simulink model "power_PVarray_grid_det"  (R2016a)
settings: Solver=FixedStepDiscrete  SolverMode=SingleTasking  StartTime=0.0  StopTime=2.5  RelTol=1e-3
PreLoadFcn:
  | Ts_Power=1e-6;
  | Ts_Control=100e-6;
undefined symbols (not defined in the file): D1, Delta, DiscIntNeverNeededParam, sigbuilder_block
libraries: powerlib x23, powerlib_meascontrol x11, simulink x2, re_lib x1
(part 1 of 2)
Description:
  | Copyright 2008-2016 The MathWorks, Inc.
settings Model: SimulationMode=accelerator  Creator=MathWorks  LastModifiedBy=mesutto
settings DataIOCC: LimitDataPoints=on  SaveFormat=Array  SignalLoggingSaveFormat=ModelDataLogs  SignalLogging=off  DSMLogging=off
settings OptimizationCC: ExpressionDepthLimit=2147483647
settings DebuggingCC: UnderspecifiedInitializationDetection=Classic  MergeDetectMultiDrivingBlocksExec=none  SolverPrmCheckMsg=warning  FcnCallInpInsideContextMsg=UseLocalSettings  StateNameClashWarn=warning
settings HardwareCC: ProdBitPerPointer=32  ProdLargestAtomicFloat=None  ProdIntDivRoundTo=Undefined  ProdEndianess=Unspecified  ProdWordSize=32  ProdHWDeviceType=32-bit Generic
settings ModelReferenceCC: PropagateSignalLabelsOutOfModel=off
settings GRTTargetCC: CombineOutputUpdateFcns=off  GRTInterface=on
settings ConfigComp: CovModelRefEnable=Off  CovSFcnEnable=off

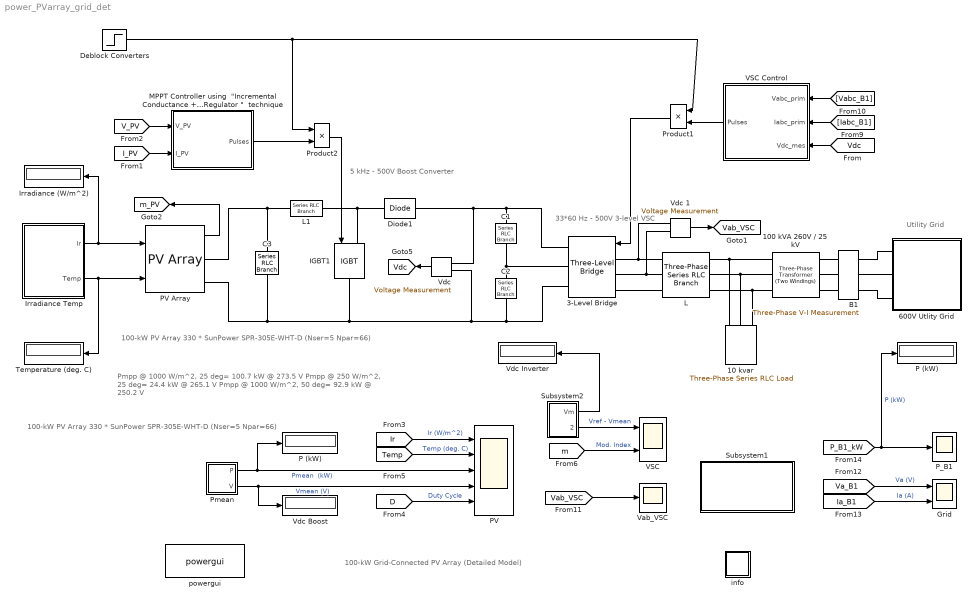
== system power_PVarray_grid_det ==
  note: 5 kHz - 500V
      | Boost Converter
  note: 33*60 Hz - 500V
      | 3-level VSC
  note: 100-kW Grid-Connected PV Array (Detailed Model)
  note: Utility Grid
  note: Pmpp @ 1000 W/m^2, 25 deg= 100.7 kW @ 273.5 V
      | Pmpp @  250 W/m^2, 25 deg= 24.4  kW @ 265.1 V
      | Pmpp @ 1000 W/m^2, 50 deg= 92.9  kW @ 250.2 V
  note: 100-kW  PV Array
      | 330 * SunPower SPR-305E-WHT-D  (Nser=5 Npar=66)
  note: 100-kW  PV Array
      | 330 * SunPower SPR-305E-WHT-D  (Nser=5 Npar=66)
  10 kvar : powerlib/Elements/Three-Phase Series RLC Load  LConnTagsString=A|B|C  Configuration=Y (grounded)  NominalVoltage=240  Vabc=[1e3 1e3 1e3]  Vabcp=[1e3 1e3 1e3]  NominalFrequency=60  UnbalancedPower=off  ActivePower=10e3/100  InductivePower=0  CapacitivePower=10e3  Pabc=[10e3 9e3 11e3]  QLabc=[100 90 110]  QCabc=[100 90 110]  Pabcp=[10e3 9e3 11e3]  QLabcp=[100 90 110]  QCabcp=[100 90 110]  Measurements=None  LoadType=constant Z
  100 kVA 260V / 25 kV : powerlib/Elements/Three-Phase Transformer (Two Windings)  Winding1Connection=Yg  Winding2Connection=Delta (D1)  CoreType=Three single-phase transformers  SetSaturation=off  Hysteresis=off  DataFile='hysteresis'  SetInitialFlux=off  Measurements=None  UNITS=pu  NominalPower=[100e3 , 60 ]  Winding1=[ 25e3 , 0.001 , 0.03 ]  Winding2=[ 260 , 0.001 , 0.03 ]  Rm=500  Lm=500  L0=0.5  Saturation=[ 0,0 ; 0.0024,1.2 ; 1.0,1.52 ]  InitialFluxes=[ 0.8 , -0.8 , 0.7 ]  MoreParameters=off  BreakLoop=off  DataType=off  TransfoNumber=0
  3-Level Bridge : powerlib/Power Electronics/Three-Level Bridge  Arms=3  SnubberResistance=1e6  SbubberCapacitance=inf  Device=IGBT / Diodes  Ron=0.2e-3  ForwardVoltages="[  0  0 ]"  Measurements=None
  600V Utlity Grid : Subsystem
      mask Display: image(imread('grid.jpg'))
  B1 : powerlib/Measurements/Three-Phase V-I Measurement  VoltageMeasurement=phase-to-ground  SetLabelV=on  LabelV=Vabc_B1  Vpu=off  VpuLL=off  CurrentMeasurement=yes  SetLabelI=on  LabelI=Iabc_B1  Ipu=off  Pbase=100e6  Vbase=500e3  OutputType=Magnitude  PhasorSimulation=off  PSBequivalent=0
  C1 : powerlib/Elements/Series RLC Branch  LConnTagsString=__new0  RConnTagsString=__new0  BranchType=C  Resistance=1.0  Inductance=1.0  SetiL0=off  InitialCurrent=0  Capacitance=12000e-06  Setx0=off  InitialVoltage=0  Measurements=None
  C2 : powerlib/Elements/Series RLC Branch  LConnTagsString=__new0  RConnTagsString=__new0  BranchType=C  Resistance=1.0  Inductance=1.0  SetiL0=off  InitialCurrent=0  Capacitance=12000e-06  Setx0=off  InitialVoltage=0  Measurements=None
  C3 : powerlib/Elements/Series RLC Branch  LConnTagsString=__new0  RConnTagsString=__new0  BranchType=C  Resistance=1.0  Inductance=1.0  SetiL0=off  InitialCurrent=0  Capacitance=100e-6  Setx0=off  InitialVoltage=0  Measurements=Branch voltage
  Deblock Converters : Step  Time=0.05  SampleTime=0
  Diode1 : powerlib/Power Electronics/Diode  Ron=1e-4  Lon=0  Vf=0  IC=0  UseSnubber=off  Rs=inf  Cs=inf  Measurements=off
  Grid : Scope  NumInputPorts=2
  IGBT1 : powerlib/Power Electronics/IGBT  Ron=0.001  Lon=0  Vf=0  Tf=0  Tt=0  IC=0  Rs=1e5  Cs=inf  Measurements=off
  Irradiance (W/m^2) : Display
      settings: Format=bank  Decimation=1000
  Irradiance Temp : Subsystem  Tag=STV Subsys  LoadFcn=sigbuilder_block('load');  StartFcn=sigbuilder_block('start');  StopFcn=sigbuilder_block('stop');  ClipboardFcn=sigbuilder_block('clipboard');  mask(Sigbuilder block){}
      mask help: Sigbuilder GUI
      mask init:
      | if ~strcmp(get_param(bdroot(gcbh),'SimulationStatus'),'stopped') tuvar = sigbuilder_block('maskInit'); end
      settings: CopyFcn=sigbuilder_block('copy');  DeleteFcn=sigbuilder_block('delete');  ModelCloseFcn=sigbuilder_block('modelClose');  PreSaveFcn=sigbuilder_block('preSave');  PauseFcn=sigbuilder_block('pause')  ContinueFcn=sigbuilder_block('continue')  NameChangeFcn=sigbuilder_block('namechange');  OpenFcn=sigbuilder_block('open',[216.75 153.75 550.5 395.25 ]);  CloseFcn=sigbuilder_block('close');
      mask Display: plot(0,0,100,100,[10,10,40,40,10],[80,20,20,80,80],[40,10],[50,50], [40,27,10],[65,72,56],[40,25,25,10],[28,28,43,43]);
  L : powerlib/Elements/Three-Phase Series RLC Branch  LConnTagsString=A|B|C  RConnTagsString=A|B|C  BranchType=RL  Resistance=500e-6*377/50/2  Inductance=500e-6/2  Capacitance=inf  Measurements=None
  L1 : powerlib/Elements/Series RLC Branch  LConnTagsString=__new0  RConnTagsString=__new0  BranchType=RL  Resistance=0.005  Inductance=5e-3  SetiL0=off  InitialCurrent=0  Capacitance=1e-6  Setx0=off  InitialVoltage=0  Measurements=None
  "MPPT Controller using  \"Incremental Conductance + Integral Regulator \"  technique " : Subsystem  mask(Boost Control - MPPT){fc=5000, T_MPPT=200e-6, Dinit=0.5}
      mask prompts: fc "PWM switching frequency (Hz)"; T_MPPT "Time window used by MPPT control (s)"; Dinit "Initial value of duty cycle"
  P (kW) : Display
      settings: Format=bank  Decimation=2000
  "P (kW) " : Display
      settings: Format=bank  Decimation=2000
  PV : Scope  NumInputPorts=5
  PV Array : re_lib/Solar/PV Array  Npar=66  Nser=5  PlotType=array @ 1000 W/m2 & specified temperatures  S_vec="[ 1000  250 ]"  Temp_C_vec="[0 25 50  ]"  ModuleName=SunPower SPR-305E-WHT-D  PlotWhenSelected=off  Pm=305.226  Ncell=96  Voc=64.2  Isc=5.96  Vm=54.7  Im=5.58  beta_Voc_pc=-0.27269  alpha_Isc_pc=0.061745  beta_Voc=-0.17507  alpha_Isc=0.00368  IL=6.0092  I0=6.3014e-12  nI=0.94504  Rsh=269.5934  Rs=0.37152  BAL=on  Tc=Tc  Tfilter=5e-5
  P_B1 : Scope
  Pmean : Subsystem
  Product1 : Product  RndMeth=Zero
  Product2 : Product  RndMeth=Zero
  Subsystem1 : Subsystem
      mask Display: disp('Open this block\nto display additional \nscopes & measurements')
  Subsystem2 : Subsystem
  Temperature (deg. C) : Display
      settings: Format=bank  Decimation=1000
  VSC : Scope  NumInputPorts=2
  VSC Control : Subsystem  mask(VSC Main Controller){nom=[ 100e3  60 ], Vnom=[ 25e3 260 ], Vnom_dc=500, RLxfo=[0.002  0.06 ], RLchoke=[2e-3  250e-6  ], K_VDCreg=[7  800], K_Ireg=[0.3 20], Ts=Ts_Control}
      mask prompts: nom "Nominal power and frequency [ Pnom(VA)  Fnom(Hz) ]:"; Vnom "Nominal primary and secondary voltages (Vrms LL) [ Vnom_prim   Vnom_sec ]:"; Vnom_dc "Nominal DC bus voltage (V):"; RLxfo "Total transformer leakage impedance (pu/Pnom) [ Rxfo  Lxf ]"; RLchoke "Choke impedance [ R(ohm) L(H) ]"; K_VDCreg "VDC regultator gains [ Kp  Ki ]:"; K_Ireg "Current regulator gains [ Kp  Ki ]:"; Ts "Sample time"
      mask init:
      | Pnom=nom(1);
      | Fnom=nom(2);
      | Vnom_prim=Vnom(1);
      | Vnom_sec=Vnom(2);
      | Zbase=Vnom_sec^2/Pnom;
      | Rtot_pu=RLxfo(1) + RLchoke(1)/Zbase;
      | Ltot_pu=RLxfo(2) + RLchoke(2)/(Zbase/(2*pi*Fnom));
      | Kp_VDCreg=K_VDCreg(1);
      | Ki_VDCreg=K_VDCreg(2);
      | Kp_Ireg=K_Ireg(1);
      | Ki_Ireg=K_Ireg(2);
      | Vdc_ref=Vnom_dc;
      | % Used to determine initial value of Boost Control (MPPT)
      | assignin('base','Vdc_ref_Inv',Vdc_ref);
  Vab_VSC : Scope
  "Vdc " : powerlib/Measurements/Voltage Measurement  Tag=PoWeRsYsTeMmEaSuReMeNt  PhasorSimulation=off  OutputType=Magnitude  PSBequivalent=0
  Vdc 1 : powerlib/Measurements/Voltage Measurement  Tag=PoWeRsYsTeMmEaSuReMeNt  PhasorSimulation=off  OutputType=Magnitude  PSBequivalent=0
  Vdc Boost : Display
      settings: Format=bank  Decimation=2000
  Vdc Inverter : Display
      settings: Format=bank  Decimation=2000
  info : Subsystem
      settings: OpenFcn=showdemo(bdroot(gcb))
      mask Display: disp('?')
  powergui : powerlib/powergui  Priority=1  SimulationMode=Discrete  SolverType=Tustin/Backward Euler (TBE)  SampleTime=Ts_Power  frequency=60  SPID=off  DisableSnubberDevices=off  DisableRonSwitches=off  DisableVfSwitches=off  SwTol=0  DisplayEquations=off  Interpol=off  ExternalGateDelay=off  methode=off  Ts=0  FunctionMessages=off  echomessages=off  HookPort=off  EnableUseOfTLC=off  x0status=blocks  frequencyindice=0  Pbase=100e6  ErrMax=1e-4  Iterations=50  UnitsV=kV  UnitsW=MW  buscounter=0  RestoreLinks=warning  ResistiveCurrentMeasurement=off  Frange=[0:2:500]  Ylog=off  Xlog=on  ShowGrid=off  save=off  variable=ZData  structure=0  ZoomFFT=on  StartTime=0.0  cycles=1  DisplayStyle=1  fundamental=60  FreqAxis=off  MaxFrequency=1000  frequencyindicesteady=1  RmsSteady=1  display=off
  tag scope: Vab_VSC=global, Vdc=global, m_PV=global
  wires:
  "Vdc "/1 -> [Vdc]
  Product2/1 -> IGBT1/1
  "MPPT Controller using  \"Incremental Conductance + Integral Regulator \"  technique "/1(Pulses) -> Product2/2
  Deblock Converters/1 -> Product2/1, Product1/1
  [Vabc_B1] -> VSC Control/1(Vabc_prim)
  [Iabc_B1] -> VSC Control/2(Iabc_prim)
  [Vdc] -> VSC Control/3(Vdc_mes)
  VSC Control/1(Pulses) -> Product1/2
  Product1/1 -> 3-Level Bridge/1
  [I_PV] -> "MPPT Controller using  \"Incremental Conductance + Integral Regulator \"  technique "/2(I_PV)
  [V_PV] -> "MPPT Controller using  \"Incremental Conductance + Integral Regulator \"  technique "/1(V_PV)
  Pmean/1(P) -> "P (kW) "/1, PV/3  "Pmean  (kW)"
  [m] -> VSC/2  "Mod. Index"
  Vdc 1/1 -> [Vab_VSC]
  [Vab_VSC] -> Vab_VSC/1
  [Ia_B1] -> Grid/2  "Ia (A)"
  [Va_B1] -> Grid/1  "Va (V)"
  [P_B1_kW] -> P_B1/1, P (kW)/1  "P (kW)"
  Pmean/2(V) -> Vdc Boost/1, PV/4  "Vmean (V)"
  Subsystem2/2(VrVm) -> VSC/1  "Vref - Vmean"
  Subsystem2/1(Vm) -> Vdc Inverter/1
  PV Array/1 -> [m_PV]
  Irradiance Temp/1(Ir) -> PV Array/1, Irradiance (W/m^2)/1
  Irradiance Temp/2(Temp) -> PV Array/2, Temperature (deg. C)/1
  [D] -> PV/5  "Duty Cycle"
  [Temp] -> PV/2  "Temp (deg. C)"
  [Ir] -> PV/1  "Ir (W/m^2)"
  connections:
  3-Level Bridge/RConn1 -- Diode1/RConn1 -- "Vdc "/LConn1 -- C1/LConn1
  L1/RConn1 -- Diode1/LConn1 -- IGBT1/LConn1
  3-Level Bridge/RConn3 -- C2/RConn1 -- "Vdc "/LConn2 -- IGBT1/RConn1 -- PV Array/RConn2 -- C3/RConn1
  3-Level Bridge/LConn1 -- L/LConn1 -- Vdc 1/LConn1
  3-Level Bridge/LConn2 -- L/LConn2 -- Vdc 1/LConn2
  3-Level Bridge/LConn3 -- L/LConn3
  L/RConn1 -- 100 kVA 260V / 25 kV/RConn1 -- 10 kvar/LConn1
  L/RConn2 -- 100 kVA 260V / 25 kV/RConn2 -- 10 kvar/LConn2
  L/RConn3 -- 100 kVA 260V / 25 kV/RConn3 -- 10 kvar/LConn3
  B1/LConn1 -- 100 kVA 260V / 25 kV/LConn1
  B1/LConn2 -- 100 kVA 260V / 25 kV/LConn2
  B1/LConn3 -- 100 kVA 260V / 25 kV/LConn3
  C2/LConn1 -- C1/RConn1 -- 3-Level Bridge/RConn2
  C3/LConn1 -- PV Array/RConn1 -- L1/LConn1
  B1/RConn2 -- 600V Utlity Grid/LConn2
  B1/RConn1 -- 600V Utlity Grid/LConn1
  B1/RConn3 -- 600V Utlity Grid/LConn3

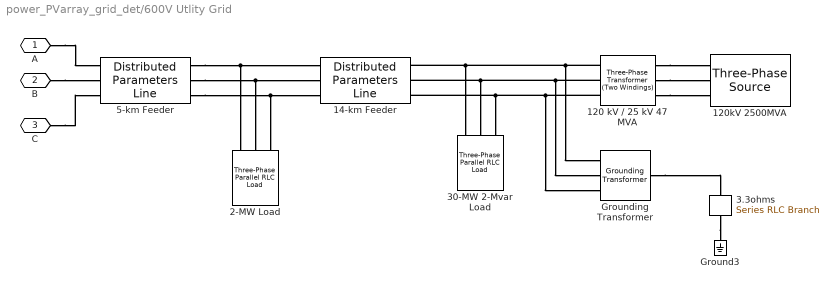
== system power_PVarray_grid_det/600V Utlity Grid ==
  120 kV / 25 kV 47 MVA : powerlib/Elements/Three-Phase Transformer (Two Windings)  Winding1Connection=Yg  Winding2Connection=Delta (D1)  CoreType=Three single-phase transformers  SetSaturation=off  Hysteresis=off  DataFile='basic_model'  SetInitialFlux=off  Measurements=None  UNITS=pu  NominalPower=[47e6 60 ]  Winding1="[ 120e3  0.08/30   0.08 ]"  Winding2="[ 25e3  0.08/30  0.08]"  Rm=500  Lm=500  L0=0.5  Saturation="[ 0,0  ;  0.005,1.2  ;  1.0,1.4 ]"  InitialFluxes=[ 0.8 , -0.8 , 0.7 ]  MoreParameters=off  BreakLoop=off  DataType=off  TransfoNumber=0
  120kV 2500MVA : powerlib/Electrical Sources/Three-Phase Source  InternalConnection=Yg  VoltagePhases=off  Voltage=120e3  PhaseAngle=0  Voltage_phases=[25e3 25e3 25e3]/sqrt(3)  PhaseAngles_phases=[0 -120 +120]  Frequency=60  NonIdealSource=on  SpecifyImpedance=on  Resistance=0.8929  Inductance=16.58e-3  ShortCircuitLevel=2500e6  BaseVoltage=120e3  XRratio=7  BusType=swing  Pref=0  Qref=0  Prefabc=[10e3, 10e3, 10e3]  Qrefabc=[0, 0, 0]  Qmin=-inf  Qmax=inf
  14-km Feeder : powerlib/Elements/Distributed Parameters Line  Phases=3  Frequency=60  Resistance=[0.1153 0.413]  Inductance=[1.05e-3 3.32e-3]  Capacitance=[11.33e-009 5.01e-009]  Length=14  x1=[-5.8e-05 -3.03124509742695e-09 0 0;-5.7e-05 -3.03083569384269e-09 0 0;-5.6e-05 -3.03042585950908e-09 0 0;-5.5e-05 -3.03001559448437e-09 0 0;-5.4e-05 -3.02960489882688e-09 0 0;-5.3e-05 -3.02919377259496e-09 0 0;-5.2e-05 -3.02878221584705e-09 0 0;-5.1e-05 -3.02837022864164e-09 0 0;-5e-05 -3.02795781103729e-09 0 0;-4.9e-05 -3.0275449630926e-09 -3790.73535189758 -24061.413420025;-4.8e-05 -3.02713168486625e-09 -3781.66414358219 -24062.8407837194;-4.7e-05 -3.02671797641698e-09 -3772.59239780798 -24064.2647275475;-4.6e-05 -3.02630383780358e-09 -3763.52011586426 -24065.6852513069;-4.5e-05 -3.02588926908492e-09 -3754.4472990404 -24067.1023547957;-4.4e-05 -3.02547427031991e-09 -3745.37394862584 -24068.5160378125;-4.3e-05 -3.02505884156753e-09 -3736.30006591012 -24069.9263001565;-4.2e-05 -3.02464298288683e-09 -3727.22565218283 -24071.3331416271;-4.1e-05 -3.0242266943369e-09 -3718.15070873366 -24072.7365620244;-4e-05 -3.02380997597692e-09 -3709.07523685235 -24074.136561149;-3.9e-05 -3.0233928278661e-09 -3699.99923782873 -24075.5331388019;-3.8e-05 -3.02297525006373e-09 -3690.9227129527 -24076.9262947847;-3.7e-05 -3.02255724262917e-09 -3681.84566351424 -24078.3160288992;-3.6e-05 -3.02213880562181e-09 -3672.7680908034 -24079.7023409481;-3.5e-05 -3.02171993910113e-09 -3663.6899961103 -24081.0852307342;-3.4e-05 -3.02130064312665e-09 -3654.61138072515 -24082.4646980611;-3.3e-05 -3.02088091775798e-09 -3645.53224593822 -24083.8407427326;-3.2e-05 -3.02046076305475e-09 -3636.45259303985 -24085.2133645533;-3.1e-05 -3.02004017907669e-09 -3627.37242332048 -24086.582563328;-3e-05 -3.01961916588357e-09 -3618.29173807058 -24087.9483388622;-2.9e-05 -3.01919772353522e-09 -3609.21053858074 -24089.3106909617;-2.8e-05 -3.01877585209154e-09 -3600.12882614158 -24090.6696194329;-2.7e-05 -3.01835355161249e-09 -3591.04660204383 -24092.0251240827;-2.6e-05 -3.01793082215809e-09 -3581.96386757827 -24093.3772047185;-2.5e-05 -3.01750766378841e-09 -3572.88062403577 -24094.725861148;-2.4e-05 -3.0170840765636e-09 -3563.79687270724 -24096.0710931796;-2.3e-05 -3.01666006054385e-09 -3554.7126148837 -24097.4129006222;-2.2e-05 -3.01623561578943e-09 -3545.62785185622 -24098.7512832849;-2.1e-05 -3.01581074236066e-09 -3536.54258491595 -24100.0862409777;-2e-05 -3.01538544031793e-09 -3527.45681535411 -24101.4177735107;-1.9e-05 -3.01495970972168e-09 -3518.37054446199 -24102.7458806947;-1.8e-05 -3.01453355063242e-09 -3509.28377353094 -24104.0705623411;-1.7e-05 -3.01410696311071e-09 -3500.19650385241 -24105.3918182614;-1.6e-05 -3.01367994721718e-09 -3491.1087367179 -24106.709648268;-1.5e-05 -3.01325250301252e-09 -3482.02047341897 -24108.0240521735;-1.4e-05 -3.01282463055748e-09 -3472.93171524728 -24109.3350297911;-1.3e-05 -3.01239632991286e-09 -3463.84246349455 -24110.6425809346;-1.2e-05 -3.01196760113955e-09 -3454.75271945255 -24111.9467054181;-1.1e-05 -3.01153844429847e-09 -3445.66248441314 -24113.2474030561;-1e-05 -3.01110885945062e-09 -3436.57175966825 -24114.544673664;-9e-06 -3.01067884665704e-09 -3427.48054650987 -24115.8385170572;-8e-06 -3.01024840597885e-09 -3418.38884623006 -24117.128933052;-7e-06 -3.00981753747724e-09 -3409.29666012097 -24118.4159214649;-6e-06 -3.00938624121342e-09 -3400.20398947478 -24119.6994821131;-5e-06 -3.00895451724871e-09 -3391.11083558378 -24120.979614814;-4e-06 -3.00852236564446e-09 -3382.0171997403 -24122.2563193858;-3e-06 -3.00808978646208e-09 -3372.92308323675 -24123.5295956469;-2e-06 -3.00765677976306e-09 -3363.82848736562 -24124.7994434166;-1e-06 -3.00722334560893e-09 -3354.73341341943 -24126.0658625142]  x2=[-5.8e-05 -3.18873630316946e-09 0 0;-5.7e-05 -3.18824656390701e-09 0 0;-5.6e-05 -3.18775637152362e-09 0 0;-5.5e-05 -3.18726572608896e-09 0 0;-5.4e-05 -3.18677462767275e-09 0 0;-5.3e-05 -3.1862830763448e-09 0 0;-5.2e-05 -3.18579107217497e-09 0 0;-5.1e-05 -3.18529861523317e-09 0 0;-5e-05 -3.18480570558941e-09 0 0;-4.9e-05 -3.18431234331373e-09 -3379.39242591108 -24244.0512732151;-4.8e-05 -3.18381852847625e-09 -3370.25239397928 -24245.323551305;-4.7e-05 -3.18332426114715e-09 -3361.11188305945 -24246.5923835937;-4.6e-05 -3.18282954139668e-09 -3351.97089445066 -24247.8577699009;-4.5e-05 -3.18233436929515e-09 -3342.82942945205 -24249.1197100467;-4.4e-05 -3.18183874491293e-09 -3333.68748936283 -24250.3782038519;-4.3e-05 -3.18134266832047e-09 -3324.54507548227 -24251.6332511374;-4.2e-05 -3.18084613958826e-09 -3315.40218910972 -24252.884851725;-4.1e-05 -3.18034915878689e-09 -3306.25883154457 -24254.1330054368;-4e-05 -3.17985172598696e-09 -3297.11500408631 -24255.3777120954;-3.9e-05 -3.1793538412592e-09 -3287.97070803447 -24256.6189715239;-3.8e-05 -3.17885550467434e-09 -3278.82594468867 -24257.8567835459;-3.7e-05 -3.17835671630323e-09 -3269.68071534858 -24259.0911479854;-3.6e-05 -3.17785747621674e-09 -3260.53502131394 -24260.3220646671;-3.5e-05 -3.17735778448583e-09 -3251.38886388456 -24261.5495334159;-3.4e-05 -3.17685764118153e-09 -3242.24224436031 -24262.7735540575;-3.3e-05 -3.1763570463749e-09 -3233.09516404113 -24263.9941264179;-3.2e-05 -3.1758560001371e-09 -3223.94762422702 -24265.2112503236;-3.1e-05 -3.17535450253933e-09 -3214.79962621806 -24266.4249256016;-3e-05 -3.17485255365287e-09 -3205.65117131437 -24267.6351520794;-2.9e-05 -3.17435015354906e-09 -3196.50226081616 -24268.841929585;-2.8e-05 -3.1738473022993e-09 -3187.35289602369 -24270.045257947;-2.7e-05 -3.17334399997506e-09 -3178.20307823729 -24271.2451369943;-2.6e-05 -3.17284024664786e-09 -3169.05280875736 -24272.4415665564;-2.5e-05 -3.17233604238931e-09 -3159.90208888435 -24273.6345464632;-2.4e-05 -3.17183138727105e-09 -3150.75091991877 -24274.8240765452;-2.3e-05 -3.17132628136482e-09 -3141.59930316123 -24276.0101566333;-2.2e-05 -3.17082072474239e-09 -3132.44723991236 -24277.192786559;-2.1e-05 -3.17031471747563e-09 -3123.29473147288 -24278.3719661542;-2e-05 -3.16980825963644e-09 -3114.14177914356 -24279.5476952513;-1.9e-05 -3.16930135129681e-09 -3104.98838422525 -24280.7199736831;-1.8e-05 -3.16879399252877e-09 -3095.83454801884 -24281.8888012832;-1.7e-05 -3.16828618340444e-09 -3086.6802718253 -24283.0541778853;-1.6e-05 -3.16777792399598e-09 -3077.52555694565 -24284.2161033239;-1.5e-05 -3.16726921437563e-09 -3068.37040468099 -24285.3745774338;-1.4e-05 -3.1667600546157e-09 -3059.21481633246 -24286.5296000503;-1.3e-05 -3.16625044478853e-09 -3050.05879320128 -24287.6811710094;-1.2e-05 -3.16574038496656e-09 -3040.90233658873 -24288.8292901473;-1.1e-05 -3.16522987522229e-09 -3031.74544779614 -24289.9739573009;-1e-05 -3.16471891562825e-09 -3022.5881281249 -24291.1151723075;-9e-06 -3.16420750625709e-09 -3013.43037887649 -24292.2529350049;-8e-06 -3.16369564718146e-09 -3004.27220135241 -24293.3872452314;-7e-06 -3.16318333847413e-09 -2995.11359685425 -24294.5181028257;-6e-06 -3.16267058020791e-09 -2985.95456668366 -24295.6455076273;-5e-06 -3.16215737245566e-09 -2976.79511214233 -24296.7694594758;-4e-06 -3.16164371529032e-09 -2967.63523453202 -24297.8899582115;-3e-06 -3.16112960878491e-09 -2958.47493515457 -24299.0070036751;-2e-06 -3.16061505301248e-09 -2949.31421531185 -24300.1205957079;-1e-06 -3.16010004804616e-09 -2940.1530763058 -24301.2307341517]  x3=[-5.8e-05 -1.72413029855508e-11 0 0;-5.7e-05 -1.72422114793655e-11 0 0;-5.6e-05 -1.72431175226773e-11 0 0;-5.5e-05 -1.72440211153576e-11 0 0;-5.4e-05 -1.72449222572779e-11 0 0;-5.3e-05 -1.72458209483102e-11 0 0;-5.2e-05 -1.72467171883267e-11 0 0;-5.1e-05 -1.72476109772001e-11 0 0;-5e-05 -1.72485023148033e-11 0 0;-4.9e-05 -1.72493912010096e-11 -23.54428473825 -155.681477773822;-4.8e-05 -1.72502776356928e-11 -23.4855925321313 -155.690342696943;-4.7e-05 -1.72511616187268e-11 -23.4268969881861 -155.699185492994;-4.6e-05 -1.7252043149986e-11 -23.3681981147565 -155.708006160718;-4.5e-05 -1.72529222293451e-11 -23.3094959201847 -155.716804698862;-4.4e-05 -1.72537988566793e-11 -23.2507904128137 -155.725581106176;-4.3e-05 -1.72546730318638e-11 -23.1920816009869 -155.734335381411;-4.2e-05 -1.72555447547744e-11 -23.133369493048 -155.743067523325;-4.1e-05 -1.72564140252873e-11 -23.0746540973415 -155.751777530675;-4e-05 -1.7257280843279e-11 -23.015935422212 -155.760465402224;-3.9e-05 -1.72581452086261e-11 -22.9572134760047 -155.769131136737;-3.8e-05 -1.7259007121206e-11 -22.8984882670655 -155.777774732983;-3.7e-05 -1.7259866580896e-11 -22.8397598037404 -155.786396189732;-3.6e-05 -1.72607235875741e-11 -22.781028094376 -155.794995505761;-3.5e-05 -1.72615781411184e-11 -22.7222931473195 -155.803572679846;-3.4e-05 -1.72624302414075e-11 -22.6635549709184 -155.812127710769;-3.3e-05 -1.72632798883202e-11 -22.6048135735207 -155.820660597314;-3.2e-05 -1.72641270817359e-11 -22.5460689634749 -155.829171338267;-3.1e-05 -1.72649718215341e-11 -22.4873211491298 -155.83765993242;-3e-05 -1.72658141075948e-11 -22.428570138835 -155.846126378567;-2.9e-05 -1.72666539397982e-11 -22.3698159409401 -155.854570675503;-2.8e-05 -1.72674913180251e-11 -22.3110585637954 -155.862992822028;-2.7e-05 -1.72683262421563e-11 -22.2522980157518 -155.871392816947;-2.6e-05 -1.72691587120733e-11 -22.1935343051604 -155.879770659064;-2.5e-05 -1.72699887276576e-11 -22.1347674403728 -155.88812634719;-2.4e-05 -1.72708162887914e-11 -22.0759974297411 -155.896459880136;-2.3e-05 -1.72716413953571e-11 -22.0172242816178 -155.904771256719;-2.2e-05 -1.72724640472373e-11 -21.9584480043559 -155.913060475756;-2.1e-05 -1.72732842443152e-11 -21.8996686063089 -155.921327536071;-2e-05 -1.72741019864742e-11 -21.8408860958305 -155.929572436487;-1.9e-05 -1.7274917273598e-11 -21.7821004812752 -155.937795175834;-1.8e-05 -1.72757301055709e-11 -21.7233117709976 -155.945995752943;-1.7e-05 -1.72765404822772e-11 -21.6645199733529 -155.954174166647;-1.6e-05 -1.72773484036018e-11 -21.6057250966968 -155.962330415786;-1.5e-05 -1.72781538694298e-11 -21.5469271493853 -155.970464499199;-1.4e-05 -1.72789568796469e-11 -21.4881261397749 -155.978576415731;-1.3e-05 -1.72797574341389e-11 -21.4293220762226 -155.986666164228;-1.2e-05 -1.7280555532792e-11 -21.3705149670857 -155.994733743541;-1.1e-05 -1.72813511754927e-11 -21.311704820722 -156.002779152524;-1e-05 -1.7282144362128e-11 -21.2528916454897 -156.010802390033;-9e-06 -1.72829350925852e-11 -21.1940754497476 -156.018803454927;-8e-06 -1.72837233667519e-11 -21.1352562418548 -156.02678234607;-7e-06 -1.7284509184516e-11 -21.0764340301706 -156.034739062328;-6e-06 -1.7285292545766e-11 -21.0176088230551 -156.042673602569;-5e-06 -1.72860734503903e-11 -20.9587806288687 -156.050585965666;-4e-06 -1.72868518982781e-11 -20.8999494559722 -156.058476150495;-3e-06 -1.72876278893187e-11 -20.8411153127267 -156.066344155934;-2e-06 -1.72884014234019e-11 -20.782278207494 -156.074189980865;-1e-06 -1.72891725004176e-11 -20.723438148636 -156.082013624173]  x4=[-5.8e-05 9.36608461567975e-12 0 0;-5.7e-05 9.36843006027392e-12 0 0;-5.6e-05 9.37077417340526e-12 0 0;-5.5e-05 9.3731169547406e-12 0 0;-5.4e-05 9.37545840394698e-12 0 0;-5.3e-05 9.37779852069164e-12 0 0;-5.2e-05 9.38013730464198e-12 0 0;-5.1e-05 9.38247475546562e-12 0 0;-5e-05 9.38481087283036e-12 0 0;-4.9e-05 9.38714565640417e-12 -1.35581366009439 -2.15298522698326;-4.8e-05 9.38947910585523e-12 -1.35500190745925 -2.15349620368565;-4.7e-05 9.39181122085192e-12 -1.35418996224812 -2.1540068743282;-4.6e-05 9.39414200106277e-12 -1.3533778245764 -2.15451723883834;-4.5e-05 9.39647144615654e-12 -1.35256549455951 -2.15502729714353;-4.4e-05 9.39879955580216e-12 -1.35175297231289 -2.15553704917128;-4.3e-05 9.40112632966876e-12 -1.35094025795203 -2.15604649484915;-4.2e-05 9.40345176742564e-12 -1.35012735159244 -2.15655563410472;-4.1e-05 9.40577586874231e-12 -1.34931425334963 -2.15706446686564;-4e-05 9.40809863328847e-12 -1.34850096333918 -2.1575729930596;-3.9e-05 9.410420060734e-12 -1.34768748167667 -2.15808121261431;-3.8e-05 9.41274015074896e-12 -1.34687380847771 -2.15858912545756;-3.7e-05 9.41505890300364e-12 -1.34605994385794 -2.15909673151715;-3.6e-05 9.41737631716846e-12 -1.34524588793304 -2.15960403072095;-3.5e-05 9.4196923929141e-12 -1.3444316408187 -2.16011102299685;-3.4e-05 9.42200712991136e-12 -1.34361720263063 -2.16061770827279;-3.3e-05 9.42432052783129e-12 -1.3428025734846 -2.16112408647678;-3.2e-05 9.42663258634509e-12 -1.34198775349638 -2.16163015753684;-3.1e-05 9.42894330512417e-12 -1.34117274278176 -2.16213592138104;-3e-05 9.43125268384013e-12 -1.34035754145659 -2.16264137793751;-2.9e-05 9.43356072216475e-12 -1.33954214963672 -2.16314652713441;-2.8e-05 9.43586741977e-12 -1.33872656743804 -2.16365136889995;-2.7e-05 9.43817277632806e-12 -1.33791079497645 -2.16415590316237;-2.6e-05 9.44047679151128e-12 -1.33709483236791 -2.16466012984998;-2.5e-05 9.44277946499221e-12 -1.33627867972837 -2.1651640488911;-2.4e-05 9.44508079644358e-12 -1.33546233717382 -2.16566766021413;-2.3e-05 9.44738078553834e-12 -1.3346458048203 -2.16617096374749;-2.2e-05 9.44967943194959e-12 -1.33382908278384 -2.16667395941964;-2.1e-05 9.45197673535065e-12 -1.33301217118052 -2.1671766471591;-2e-05 9.45427269541502e-12 -1.33219507012645 -2.16767902689443;-1.9e-05 9.4565673118164e-12 -1.33137777973774 -2.16818109855422;-1.8e-05 9.45886058422866e-12 -1.33056030013056 -2.16868286206713;-1.7e-05 9.46115251232589e-12 -1.32974263142109 -2.16918431736184;-1.6e-05 9.46344309578234e-12 -1.32892477372554 -2.16968546436708;-1.5e-05 9.46573233427248e-12 -1.32810672716013 -2.17018630301163;-1.4e-05 9.46802022747095e-12 -1.32728849184115 -2.1706868332243;-1.3e-05 9.4703067750526e-12 -1.32647006788486 -2.17118705493397;-1.2e-05 9.47259197669245e-12 -1.3256514554076 -2.17168696806953;-1.1e-05 9.47487583206572e-12 -1.3248326545257 -2.17218657255995;-1e-05 9.47715834084783e-12 -1.32401366535554 -2.1726858683342;-9e-06 9.47943950271439e-12 -1.3231944880135 -2.17318485532135;-8e-06 9.48171931734118e-12 -1.32237512261602 -2.17368353345046;-7e-06 9.4839977844042e-12 -1.32155556927955 -2.17418190265066;-6e-06 9.48627490357963e-12 -1.32073582812055 -2.17467996285112;-5e-06 9.48855067454383e-12 -1.31991589925554 -2.17517771398106;-4e-06 9.49082509697338e-12 -1.31909578280104 -2.17567515596974;-3e-06 9.49309817054501e-12 -1.31827547887362 -2.17617228874646;-2e-06 9.49536989493568e-12 -1.31745498758984 -2.17666911224057;-1e-06 9.49764026982253e-12 -1.31663430906634 -2.17716562638145]  x5=5.70973484498186e-05  V1=ones(3,3)  V2=ones(3,3)  I1=ones(3,3)  I2=ones(3,3)  nHarmo=1  Measurements=None
  2-MW Load : powerlib/Elements/Three-Phase Parallel RLC Load  LConnTagsString=A|B|C  Configuration=Y (grounded)  NominalVoltage=25e3  Vabc=[1e3 1e3 1e3]  Vabcp=[1e3 1e3 1e3]  NominalFrequency=60  UnbalancedPower=off  ActivePower=2e6  InductivePower=0  CapacitivePower=0  Pabc=[10e3 9e3 11e3]  QLabc=[100 90 110]  QCabc=[100 90 110]  Pabcp=[10e3 9e3 11e3]  QLabcp=[100 90 110]  QCabcp=[100 90 110]  Measurements=None  LoadType=constant Z
  "3.3ohms " : powerlib/Elements/Series RLC Branch  LConnTagsString=__new0  RConnTagsString=__new0  BranchType=R  Resistance=3.3  Inductance=[]  SetiL0=off  InitialCurrent=0  Capacitance=[]  Setx0=off  InitialVoltage=0  Measurements=None
  30-MW 2-Mvar Load : powerlib/Elements/Three-Phase Parallel RLC Load  LConnTagsString=A|B|C  Configuration=Y (grounded)  NominalVoltage=25e3  Vabc=[1e3 1e3 1e3]  Vabcp=[1e3 1e3 1e3]  NominalFrequency=60  UnbalancedPower=off  ActivePower=30e6  InductivePower=2e6  CapacitivePower=0  Pabc=[10e3 9e3 11e3]  QLabc=[100 90 110]  QCabc=[100 90 110]  Pabcp=[10e3 9e3 11e3]  QLabcp=[100 90 110]  QCabcp=[100 90 110]  Measurements=None  LoadType=constant Z
  5-km Feeder : powerlib/Elements/Distributed Parameters Line  Phases=3  Frequency=60  Resistance=[0.1153 0.413]  Inductance=[1.05e-3 3.32e-3]  Capacitance=[11.33e-009 5.01e-009]  Length=5  x1=[-2.1e-05 -2.97117489630349e-09 -3537.1777312942 -24101.4118174689;-2e-05 -2.97075289303274e-09 -3528.09146195667 -24102.7435893523;-1.9e-05 -2.97033046755175e-09 -3519.00469119866 -24104.0719356983;-1.8e-05 -2.96990761992056e-09 -3509.91742031161 -24105.396856318;-1.7e-05 -2.96948435019926e-09 -3500.82965058701 -24106.7183510233;-1.6e-05 -2.96906065844801e-09 -3491.74138331645 -24108.0364196263;-1.5e-05 -2.96863654472702e-09 -3482.65261979156 -24109.3510619397;-1.4e-05 -2.96821200909658e-09 -3473.56336130407 -24110.6622777766;-1.3e-05 -2.96778705161701e-09 -3464.47360914575 -24111.9700669507;-1.2e-05 -2.96736167234872e-09 -3455.38336460848 -24113.2744292761;-1.1e-05 -2.96693587135215e-09 -3446.29262898416 -24114.5753645675;-1e-05 -2.96650964868783e-09 -3437.20140356481 -24115.8728726399;-9e-06 -2.96608300441633e-09 -3428.10968964248 -24117.1669533089;-8e-06 -2.96565593859829e-09 -3419.01748850931 -24118.4576063906;-7e-06 -2.9652284512944e-09 -3409.92480145751 -24119.7448317017;-6e-06 -2.96480054256542e-09 -3400.83162977934 -24121.0286290591;-5e-06 -2.96437221247216e-09 -3391.73797476716 -24122.3089982804;-4e-06 -2.96394346107549e-09 -3382.64383771337 -24123.5859391836;-3e-06 -2.96351428843636e-09 -3373.54921991045 -24124.8594515872;-2e-06 -2.96308469461576e-09 -3364.45412265095 -24126.1295353103;-1e-06 -2.96265467967475e-09 -3355.35854722749 -24127.3961901723]  x2=[-2.1e-05 -3.01581074236066e-09 -3536.54258491595 -24100.0862409777;-2e-05 -3.01538544031793e-09 -3527.45681535411 -24101.4177735107;-1.9e-05 -3.01495970972168e-09 -3518.37054446199 -24102.7458806947;-1.8e-05 -3.01453355063242e-09 -3509.28377353094 -24104.0705623411;-1.7e-05 -3.01410696311071e-09 -3500.19650385241 -24105.3918182614;-1.6e-05 -3.01367994721718e-09 -3491.1087367179 -24106.709648268;-1.5e-05 -3.01325250301252e-09 -3482.02047341897 -24108.0240521735;-1.4e-05 -3.01282463055748e-09 -3472.93171524728 -24109.3350297911;-1.3e-05 -3.01239632991286e-09 -3463.84246349455 -24110.6425809346;-1.2e-05 -3.01196760113955e-09 -3454.75271945255 -24111.9467054181;-1.1e-05 -3.01153844429847e-09 -3445.66248441314 -24113.2474030561;-1e-05 -3.01110885945062e-09 -3436.57175966825 -24114.544673664;-9e-06 -3.01067884665704e-09 -3427.48054650987 -24115.8385170572;-8e-06 -3.01024840597885e-09 -3418.38884623006 -24117.128933052;-7e-06 -3.00981753747724e-09 -3409.29666012097 -24118.4159214649;-6e-06 -3.00938624121342e-09 -3400.20398947478 -24119.6994821131;-5e-06 -3.00895451724871e-09 -3391.11083558378 -24120.979614814;-4e-06 -3.00852236564446e-09 -3382.0171997403 -24122.2563193858;-3e-06 -3.00808978646208e-09 -3372.92308323675 -24123.5295956469;-2e-06 -3.00765677976306e-09 -3363.82848736562 -24124.7994434166;-1e-06 -3.00722334560893e-09 -3354.73341341943 -24126.0658625142]  x3=[-2.1e-05 -7.83225390734921e-12 -11.1569792961237 -79.1361755515031;-2e-05 -7.83405919337593e-12 -11.1271448686731 -79.1403760099989;-1.9e-05 -7.83586336600813e-12 -11.0973088598071 -79.1445652208823;-1.8e-05 -7.8376664249894e-12 -11.0674712737659 -79.148743183558;-1.7e-05 -7.83946837006347e-12 -11.0376321147903 -79.1529098974321;-1.6e-05 -7.84126920097425e-12 -11.007791387121 -79.1570653619124;-1.5e-05 -7.8430689174658e-12 -10.9779490949991 -79.1612095764085;-1.4e-05 -7.84486751928235e-12 -10.9481052426657 -79.1653425403312;-1.3e-05 -7.84666500616827e-12 -10.9182598343624 -79.1694642530932;-1.2e-05 -7.8484613778681e-12 -10.888412874331 -79.1735747141088;-1.1e-05 -7.85025663412653e-12 -10.8585643668132 -79.1776739227936;-1e-05 -7.85205077468842e-12 -10.8287143160512 -79.1817618785652;-9e-06 -7.85384379929878e-12 -10.7988627262875 -79.1858385808426;-8e-06 -7.85563570770279e-12 -10.7690096017645 -79.1899040290463;-7e-06 -7.85742649964576e-12 -10.7391549467251 -79.1939582225986;-6e-06 -7.8592161748732e-12 -10.7092987654123 -79.1980011609233;-5e-06 -7.86100473313074e-12 -10.6794410620693 -79.2020328434457;-4e-06 -7.8627921741642e-12 -10.6495818409395 -79.2060532695929;-3e-06 -7.86457849771954e-12 -10.6197211062667 -79.2100624387936;-2e-06 -7.86636370354288e-12 -10.5898588622946 -79.2140603504778;-1e-06 -7.8681477913805e-12 -10.5599951132675 -79.2180470040775]  x4=[-2.1e-05 -1.10829285409668e-12 -12.5606324026011 -78.9000787577051;-2e-05 -1.10553142124068e-12 -12.5308868817975 -78.9048083977202;-1.9e-05 -1.10276983126401e-12 -12.5011395800755 -78.9095268236023;-1.8e-05 -1.10000808455914e-12 -12.4713905016627 -78.9142340346808;-1.7e-05 -1.0972461815186e-12 -12.4416396507872 -78.9189300302868;-1.6e-05 -1.09448412253491e-12 -12.4118870316772 -78.9236148097527;-1.5e-05 -1.09172190800061e-12 -12.3821326485612 -78.9282883724129;-1.4e-05 -1.08895953830828e-12 -12.3523765056681 -78.9329507176031;-1.3e-05 -1.08619701385052e-12 -12.3226186072268 -78.9376018446606;-1.2e-05 -1.08343433501993e-12 -12.2928589574666 -78.9422417529245;-1.1e-05 -1.08067150220917e-12 -12.2630975606169 -78.9468704417352;-1e-05 -1.07790851581088e-12 -12.2333344209076 -78.9514879104351;-9e-06 -1.07514537621776e-12 -12.2035695425687 -78.9560941583677;-8e-06 -1.0723820838225e-12 -12.1738029298304 -78.9606891848785;-7e-06 -1.06961863901783e-12 -12.1440345869232 -78.9652729893145;-6e-06 -1.06685504219649e-12 -12.1142645180778 -78.969845571024;-5e-06 -1.06409129375126e-12 -12.0844927275253 -78.9744069293574;-4e-06 -1.06132739407493e-12 -12.0547192194968 -78.9789570636662;-3e-06 -1.05856334356031e-12 -12.0249439982239 -78.9834959733039;-2e-06 -1.05579914260022e-12 -11.9951670679383 -78.9880236576254;-1e-06 -1.05303479158754e-12 -11.965388432872 -78.9925401159871]  x5=2.03919101606495e-05  V1=ones(3,3)  V2=ones(3,3)  I1=ones(3,3)  I2=ones(3,3)  nHarmo=1  Measurements=None
  Ground3 : powerlib/Elements/Ground  LConnTagsString=a
  "Grounding Transformer " : powerlib/Elements/Grounding Transformer   UNITS=pu  NominalPower="[100e6   60]"  NominalVoltage=25e3  ZeroSequenceImpedance_pu=[0.025 0.75]  MagnetizationBranch_pu=[500 500]  ZeroSequenceImpedance_SI=[0.052083 589.05]  MagnetizationBranch_SI=[1041.7 3.927e+005]  Measurements=None
  A : PMIOPort  Port=1  Side=Left
  B : PMIOPort  Port=2  Side=Left
  C : PMIOPort  Port=3  Side=Left
  connections:
  "3.3ohms "/RConn1 -- Ground3/LConn1
  120 kV / 25 kV 47 MVA/LConn1 -- 120kV 2500MVA/RConn1
  120 kV / 25 kV 47 MVA/LConn2 -- 120kV 2500MVA/RConn2
  120 kV / 25 kV 47 MVA/LConn3 -- 120kV 2500MVA/RConn3
  120 kV / 25 kV 47 MVA/RConn1 -- "Grounding Transformer "/LConn1 -- 14-km Feeder/RConn1 -- 30-MW 2-Mvar Load/LConn1
  120 kV / 25 kV 47 MVA/RConn2 -- "Grounding Transformer "/LConn2 -- 14-km Feeder/RConn2 -- 30-MW 2-Mvar Load/LConn2
  120 kV / 25 kV 47 MVA/RConn3 -- "Grounding Transformer "/LConn3 -- 14-km Feeder/RConn3 -- 30-MW 2-Mvar Load/LConn3
  5-km Feeder/RConn1 -- 14-km Feeder/LConn1 -- 2-MW Load/LConn1
  5-km Feeder/RConn2 -- 14-km Feeder/LConn2 -- 2-MW Load/LConn2
  5-km Feeder/RConn3 -- 14-km Feeder/LConn3 -- 2-MW Load/LConn3
  A/RConn1 -- 5-km Feeder/LConn1
  B/RConn1 -- 5-km Feeder/LConn2
  C/RConn1 -- 5-km Feeder/LConn3
  "Grounding Transformer "/RConn1 -- "3.3ohms "/LConn1

== system power_PVarray_grid_det/Irradiance Temp ==
  Demux : Demux  Tag=STV Demux  Outputs=2
  FromWs : FromWorkspace  Tag=STV FromWs  VariableName=tuvar  SampleTime=0
      SigBuilderData=|
      | common.afterFinalStr = 'Extrapolate'
      | common.sampleTime = '0'
      | dataSet(1).timeRange = [0 1]
      | dataSet(1).name = 'Constant Irradiance'
      | dataSet(2).timeRange = [0 1]
      | dataSet(2).name = 'Step Irradiance'
      | dataSet(3).timeRange = [0 3]
      | dataSet(3).name = 'Ramp-up/down Irradiance'
      | sbobj.Groups(1).Name = 'Constant Irradiance'
      | sbobj.Groups(1).Signals(1).Name = 'Ir'
      | sbobj.Groups(1).Signals(1).XData = [0 1]
      | sbobj.Groups(1).Signals(1).YData = [1000 1000]
      | sbobj.Groups(1).Signals(2).Name = 'Temp'
      | sbobj.Groups(1).Signals(2).XData = [0 1 1 2]
      | sbobj.Groups(1).Signals(2).YData = [0 0 1 1]
      | sbobj.Groups(1).TimeRange = [0 1]
      | sbobj.Groups(2).Name = 'Step Irradiance'
      | sbobj.Groups(2).Signals(1).Name = 'Ir'
      | sbobj.Groups(2).Signals(1).XData = [0 0.252 0.252 1]
      | sbobj.Groups(2).Signals(1).YData = [600 600 1000 1000]
      | sbobj.Groups(2).Signals(2).Name = 'Temp'
      | sbobj.Groups(2).Signals(2).XData = [0 1 1 2]
      | sbobj.Groups(2).Signals(2).YData = [0 0 1 1]
      | sbobj.Groups(2).TimeRange = [0 1]
      | sbobj.Groups(3).Name = 'Ramp-up/down Irradiance'
      | sbobj.Groups(3).Signals(1).Name = 'Ir'
      | sbobj.Groups(3).Signals(1).XData = [0 0.6 1.1 1.2 1.7 3]
      | sbobj.Groups(3).Signals(1).YData = [1000 1000 250 250 1000 1000]
      | sbobj.Groups(3).Signals(2).Name = 'Temp'
      | sbobj.Groups(3).Signals(2).XData = [0 2 2.1 3]
      | sbobj.Groups(3).Signals(2).YData = [25 25 50 50]
      | sbobj.Groups(3).TimeRange = [0 3]
  Ir : Outport  Tag=STV Outport
  Temp : Outport  Tag=STV Outport  Port=2
  wires:
  Demux/1 -> Ir/1
  FromWs/1 -> Demux/1
  Demux/2 -> Temp/1

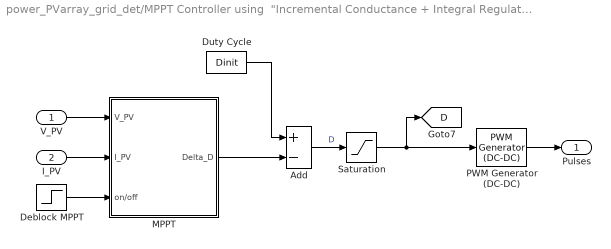
== system power_PVarray_grid_det/MPPT Controller using  "Incremental Conductance + Integral Regulator "  technique  ==
  V_PV : Inport
  I_PV : Inport  Port=2
  Add : Sum  Inputs=+-
  Deblock MPPT : Step  Time=0.4  SampleTime=0
  Duty Cycle : Constant  Value=Dinit
  MPPT : Subsystem
  PWM Generator (DC-DC) : powerlib_meascontrol/Pulse & Signal Generators/PWM Generator (DC-DC)  Fsw=fc  Ts=Ts_Power
  Saturation : Saturate  UpperLimit=1  LowerLimit=0
  Pulses : Outport
  tag scope: D=global
  wires:
  V_PV/1 -> MPPT/1(V_PV)
  I_PV/1 -> MPPT/2(I_PV)
  PWM Generator (DC-DC)/1 -> Pulses/1
  Deblock MPPT/1 -> MPPT/3(on/off)
  Saturation/1 -> PWM Generator (DC-DC)/1, [D]
  Add/1 -> Saturation/1  "D"
  MPPT/1(Delta_D) -> Add/2
  Duty Cycle/1 -> Add/1

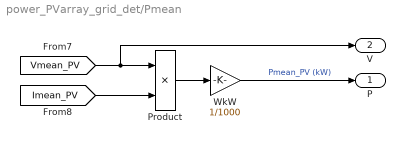
== system power_PVarray_grid_det/Pmean ==
  Product : Product  RndMeth=Zero
  WkW : Gain  Gain=1/1000
  P : Outport
  V : Outport  Port=2
  wires:
  [Vmean_PV] -> Product/1, V/1
  Product/1 -> WkW/1
  [Imean_PV] -> Product/2
  WkW/1 -> P/1  "Pmean_PV (kW)"

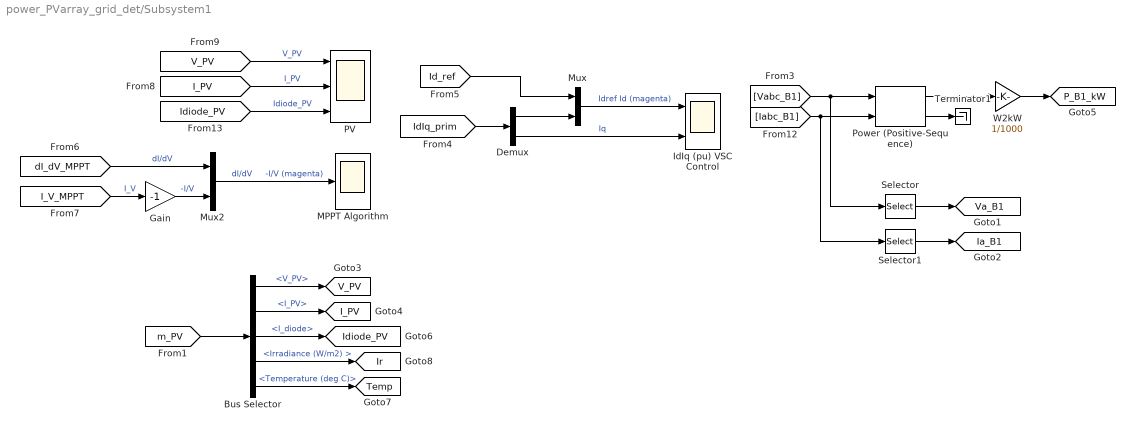
== system power_PVarray_grid_det/Subsystem1 ==
  Bus Selector : BusSelector  OutputSignals=V_PV,I_PV,I_diode,Irradiance (W/m2) ,Temperature (deg C)
  Demux : Demux  Outputs=2
  Gain : Gain  Gain=-1
  IdIq (pu) VSC Control : Scope  NumInputPorts=2
  MPPT Algorithm : Scope
  Mux : Mux  Inputs=2
  Mux2 : Mux  Inputs=2
  PV : Scope  NumInputPorts=3
  Power (Positive-Sequence) : powerlib_meascontrol/Measurements/Power (Positive-Sequence)  Freq=60  Vinit=[0, 0]  Iinit=[0, 0]  Ts=Ts_Control
  Selector : Selector  InputPortWidth=3  IndexOptions=Index vector (dialog)  Indices=[1]  OutputSizes=1
  Selector1 : Selector  InputPortWidth=3  IndexOptions=Index vector (dialog)  Indices=[1]  OutputSizes=1
  Terminator1 : Terminator
  W2kW : Gain  Gain=1/1000
  tag scope: I_PV=global, Ia_B1=global, Idiode_PV=global, Ir=global, P_B1_kW=global, Temp=global, V_PV=global, Va_B1=global
  wires:
  [Vabc_B1] -> Power (Positive-Sequence)/1, Selector/1
  [Iabc_B1] -> Power (Positive-Sequence)/2, Selector1/1
  Power (Positive-Sequence)/1 -> W2kW/1
  [I_V_MPPT] -> Gain/1  "I_V"
  [IdIq_prim] -> Demux/1
  [Id_ref] -> Mux/1
  Demux/1 -> Mux/2
  Mux/1 -> IdIq (pu) VSC Control/1  "Idref Id (magenta)"
  Demux/2 -> IdIq (pu) VSC Control/2  "Iq"
  Selector/1 -> [Va_B1]
  Selector1/1 -> [Ia_B1]
  [V_PV] -> PV/1  "V_PV"
  [I_PV] -> PV/2  "I_PV"
  [Idiode_PV] -> PV/3  "Idiode_PV"
  [dI_dV_MPPT] -> Mux2/1  "dI/dV"
  Gain/1 -> Mux2/2  "-I/V"
  Mux2/1 -> MPPT Algorithm/1  "dI/dV     -I/V (magenta)"
  W2kW/1 -> [P_B1_kW]
  [m_PV] -> Bus Selector/1
  Bus Selector/1 -> [V_PV]  "<V_PV>"
  Bus Selector/2 -> [I_PV]  "<I_PV>"
  Bus Selector/4 -> [Ir]  "<Irradiance (W/m2) >"
  Bus Selector/3 -> [Idiode_PV]  "<I_diode>"
  Bus Selector/5 -> [Temp]  "<Temperature (deg C)>"
  Power (Positive-Sequence)/2 -> Terminator1/1

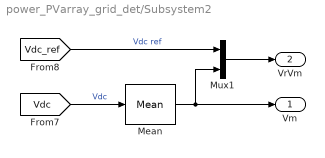
== system power_PVarray_grid_det/Subsystem2 ==
  Mean : powerlib_meascontrol/Measurements/Mean  Freq=60  Vinit=0  Ts=Ts_Control
  Mux1 : Mux  Inputs=2
  Vm : Outport
  VrVm : Outport  Port=2
  wires:
  [Vdc_ref] -> Mux1/1  "Vdc ref"
  [Vdc] -> Mean/1  "Vdc"
  Mux1/1 -> VrVm/1
  Mean/1 -> Mux1/2, Vm/1

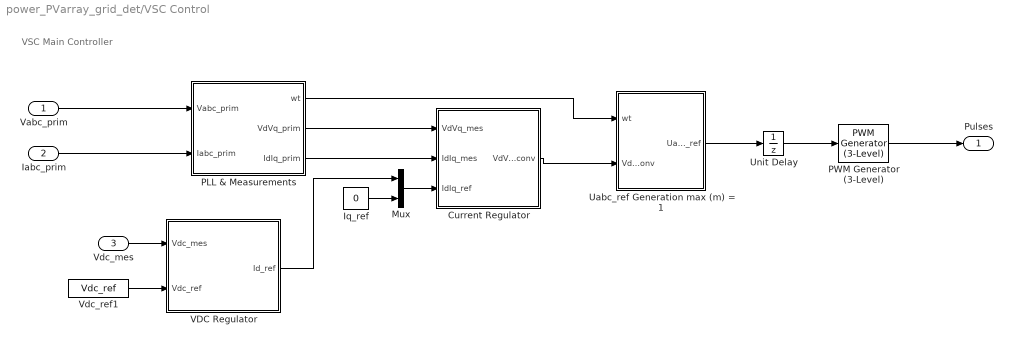
== system power_PVarray_grid_det/VSC Control ==
  note: VSC Main Controller
  Vabc_prim : Inport  PortDimensions=3
  Iabc_prim : Inport  Port=2  PortDimensions=3
  Vdc_mes : Inport  Port=3  PortDimensions=1
  Current Regulator : Subsystem
  Iq_ref : Constant  Value=0
  Mux : Mux  Inputs=2
  PLL & Measurements : Subsystem
  PWM Generator (3-Level) : powerlib_meascontrol/Pulse & Signal Generators/PWM Generator (3-Level)  ModulatorType=Three-phase bridge (12 pulses)  ModulatorMode=Unsynchronized  nF=27  Fc=33*60  ModulatingSignals=off  m=0.8  Freq=60  Phase=0  Ts=Ts_Power
  Uabc_ref Generation max (m) = 1 : Subsystem
  Unit Delay : UnitDelay  SampleTime=Ts_Control
  VDC Regulator : Subsystem
  Vdc_ref1 : Constant  Value=Vdc_ref
  Pulses : Outport
  wires:
  VDC Regulator/1(Id_ref) -> Mux/1
  PLL & Measurements/1(wt) -> Uabc_ref Generation max (m) = 1/1(wt)
  Current Regulator/1(VdVq_conv) -> Uabc_ref Generation max (m) = 1/2(VdVq_conv)
  Iq_ref/1 -> Mux/2
  Mux/1 -> Current Regulator/3(IdIq_ref)
  PLL & Measurements/3(IdIq_prim) -> Current Regulator/2(IdIq_mes)
  PLL & Measurements/2(VdVq_prim) -> Current Regulator/1(VdVq_mes)
  Vdc_mes/1 -> VDC Regulator/1(Vdc_mes)
  Vabc_prim/1 -> PLL & Measurements/1(Vabc_prim)
  Iabc_prim/1 -> PLL & Measurements/2(Iabc_prim)
  Unit Delay/1 -> PWM Generator (3-Level)/1
  PWM Generator (3-Level)/1 -> Pulses/1
  Uabc_ref Generation max (m) = 1/1(Uabc_ref) -> Unit Delay/1
  Vdc_ref1/1 -> VDC Regulator/2(Vdc_ref)

== system power_PVarray_grid_det/info ==

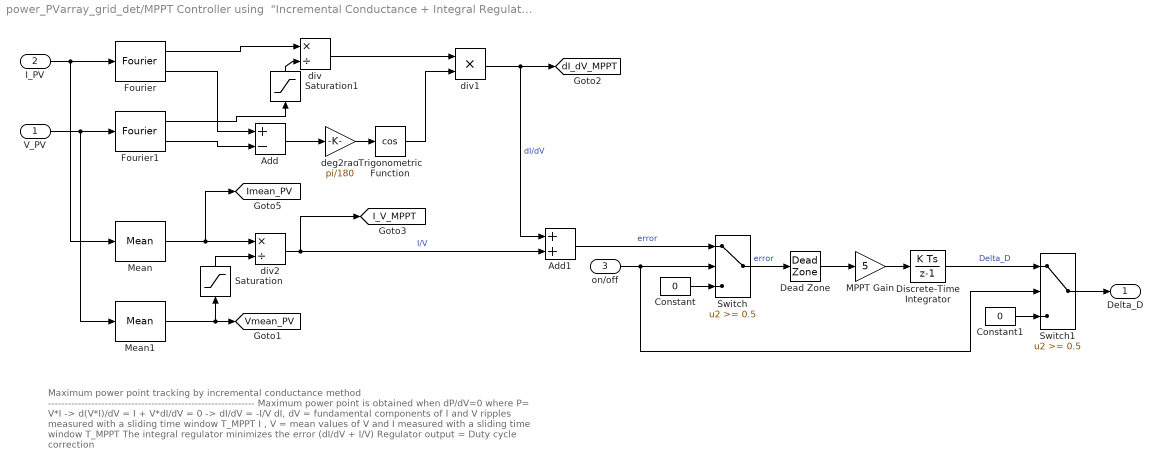
== system power_PVarray_grid_det/MPPT Controller using  "Incremental Conductance + Integral Regulator "  technique /MPPT ==
  note: Maximum power point tracking by incremental conductance method
      | --------------------------------------------------------------
      | Maximum power point is obtained when dP/dV=0  where P= V*I
      | -> d(V*I)/dV = I + V*dI/dV = 0
      | -> dI/dV = -I/V
      |
      | dI, dV  = fundamental components of I and V ripples measured with a sliding time window T_MPPT
      | I , V   = mean values of V and I measured with a sliding time window T_MPPT
      |
      | The integral regulator minimizes the error (dI/dV + I/V)
      | Regulator output = Duty cycle correction
  V_PV : Inport
  I_PV : Inport  Port=2
  on/off : Inport  Port=3
  Add : Sum  Inputs=+-
  Add1 : Sum
  Constant : Constant  Value=0
  Constant1 : Constant  Value=0
  Dead Zone : DeadZone  LowerValue=-0.05  UpperValue=0.05  SaturateOnIntegerOverflow=on
  Discrete-Time Integrator : DiscreteIntegrator  SampleTime=Ts_Control  LimitOutput=on  UpperSaturationLimit=1  LowerSaturationLimit=-1  ICPrevOutput=DiscIntNeverNeededParam  ICPrevScaledInput=DiscIntNeverNeededParam
  Fourier : powerlib_meascontrol/Measurements/Fourier  Freq=1/T_MPPT  n=1  InInit=[0, 0]  Ts=Ts_Control
  Fourier1 : powerlib_meascontrol/Measurements/Fourier  Freq=1/T_MPPT  n=1  InInit=[0, 0]  Ts=Ts_Control
  MPPT Gain : Gain  Gain=5
  Mean : powerlib_meascontrol/Measurements/Mean  Freq=1/T_MPPT  Vinit=0  Ts=Ts_Control
  Mean1 : powerlib_meascontrol/Measurements/Mean  Freq=1/T_MPPT  Vinit=0  Ts=Ts_Control
  Saturation : Saturate  UpperLimit=inf  LowerLimit=eps
  Saturation1 : Saturate  UpperLimit=inf  LowerLimit=eps
  Switch : Switch  Threshold=0.5
  Switch1 : Switch  Threshold=0.5
  Trigonometric Function : Trigonometry  Operator=cos
  deg2rad : Gain  Gain=pi/180
  div : Product  Inputs=*/  RndMeth=Zero
  div1 : Product  Inputs=**  RndMeth=Zero
  div2 : Product  Inputs=*/  RndMeth=Zero
  Delta_D : Outport
  tag scope: I_V_MPPT=global, Imean_PV=global, Vmean_PV=global, dI_dV_MPPT=global
  wires:
  Dead Zone/1 -> MPPT Gain/1
  Switch/1 -> Dead Zone/1  "error"
  Saturation1/1 -> div/2
  Saturation/1 -> div2/2
  Switch1/1 -> Delta_D/1
  on/off/1 -> Switch/2, Switch1/2
  Constant1/1 -> Switch1/3
  Discrete-Time Integrator/1 -> Switch1/1  "Delta_D"
  Constant/1 -> Switch/3
  MPPT Gain/1 -> Discrete-Time Integrator/1
  Add1/1 -> Switch/1  "error"
  div2/1 -> Add1/2, [I_V_MPPT]  "I/V"
  Mean1/1 -> Saturation/1, [Vmean_PV]
  Mean/1 -> div2/1, [Imean_PV]
  div1/1 -> Add1/1, [dI_dV_MPPT]  "dI/dV"
  Trigonometric Function/1 -> div1/2
  div/1 -> div1/1
  deg2rad/1 -> Trigonometric Function/1
  Add/1 -> deg2rad/1
  Fourier1/1 -> Saturation1/1
  Fourier1/2 -> Add/2
  Fourier/2 -> Add/1
  V_PV/1 -> Mean1/1, Fourier1/1
  I_PV/1 -> Mean/1, Fourier/1
  Fourier/1 -> div/1

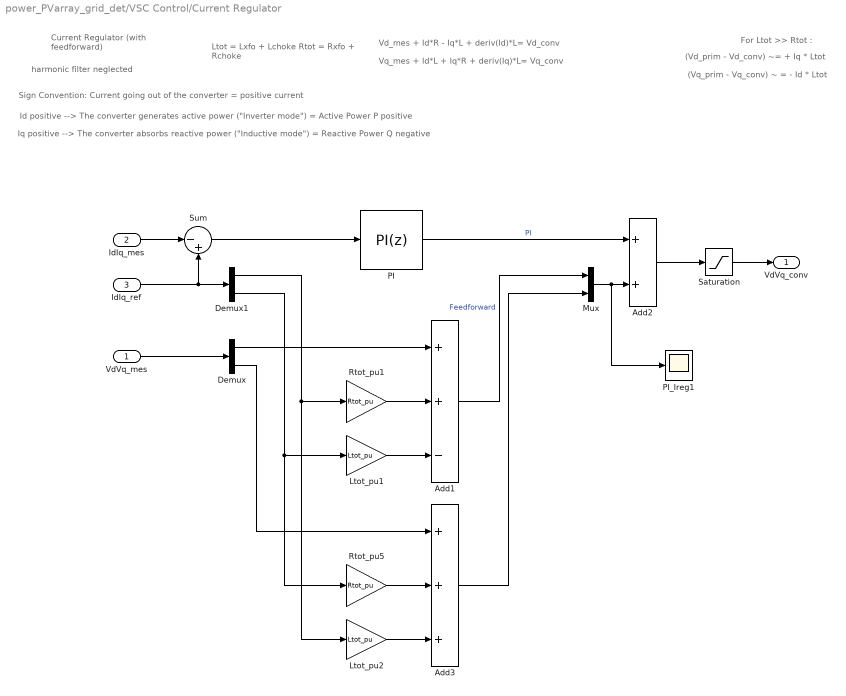
== system power_PVarray_grid_det/VSC Control/Current Regulator ==
  note: harmonic filter neglected
  note: Vd_mes + Id*R - Iq*L + deriv(Id)*L= Vd_conv
  note: Vq_mes + Id*L + Iq*R + deriv(Iq)*L= Vq_conv
  note: Current Regulator
      | (with feedforward)
  note: Sign Convention: Current going out of the converter = positive current
  note: Iq positive --> The converter absorbs reactive power ("Inductive mode") = Reactive Power Q negative
  note: Id positive --> The converter generates active power ("Inverter mode") = Active Power P positive
  note: Ltot = Lxfo + Lchoke
      | Rtot = Rxfo + Rchoke
  note: (Vd_prim - Vd_conv) ~= + Iq * Ltot
  note: (Vq_prim - Vq_conv) ~ = - Id * Ltot
  note: For Ltot >> Rtot :
  VdVq_mes : Inport  PortDimensions=2
  IdIq_mes : Inport  Port=2  PortDimensions=2
  IdIq_ref : Inport  Port=3  PortDimensions=2
  Add1 : Sum  Inputs=++-
  Add2 : Sum
  Add3 : Sum  Inputs=+++
  Demux : Demux  Outputs=2
  Demux1 : Demux  Outputs=2
  Ltot_pu1 : Gain  Gain=Ltot_pu  SaturateOnIntegerOverflow=on  OutDataTypeStr=Inherit: Same as input  ParamDataTypeStr=Inherit: Same as input
  Ltot_pu2 : Gain  Gain=Ltot_pu  SaturateOnIntegerOverflow=on  OutDataTypeStr=Inherit: Same as input  ParamDataTypeStr=Inherit: Same as input
  Mux : Mux  Inputs=2
  PI : simulink/Continuous/PID Controller  Controller=PI  TimeDomain=Discrete-time  SampleTime=Ts  IntegratorMethod=Forward Euler  FilterMethod=Forward Euler  Form=Parallel  UseFilter=on  ControllerParametersSource=internal  P=Kp_Ireg  I=Ki_Ireg  D=0  N=100  InitialConditionSource=internal  InitialConditionForIntegrator=0  InitialConditionForFilter=0  ExternalReset=none  LimitOutput=on  UpperSaturationLimit=2  LowerSaturationLimit=-2  LinearizeAsGain=off  AntiWindupMode=none  Kb=1  TrackingMode=off  Kt=1  PParamMin=[]  PParamMax=[]  IParamMin=[]  IParamMax=[]  DParamMin=[]  DParamMax=[]  NParamMin=[]  NParamMax=[]  KbParamMin=[]  KbParamMax=[]  KtParamMin=[]  KtParamMax=[]  POutMin=[]  POutMax=[]  IOutMin=[]  IOutMax=[]  DOutMin=[]  DOutMax=[]  NOutMin=[]  NOutMax=[]  KbOutMin=[]  KbOutMax=[]  KtOutMin=[]  KtOutMax=[]  IntegratorOutMin=[]  IntegratorOutMax=[]  FilterOutMin=[]  FilterOutMax=[]  SumOutMin=[]  SumOutMax=[]  SumI1OutMin=[]  SumI1OutMax=[]  SumI2OutMin=[]  SumI2OutMax=[]  SumI3OutMin=[]  SumI3OutMax=[]  SumDOutMin=[]  SumDOutMax=[]  SaturationOutMin=[]  SaturationOutMax=[]  IntegratorContinuousStateAttributes=''  IntegratorStateMustResolveToSignalObject=off  IntegratorRTWStateStorageClass=Auto  FilterContinuousStateAttributes=''  FilterStateMustResolveToSignalObject=off  FilterRTWStateStorageClass=Auto  DifferentiatorICPrevScaledInput=0  DifferentiatorOutMin=[]  DifferentiatorOutMax=[]
  PI_Ireg1 : Scope
  Rtot_pu1 : Gain  Gain=Rtot_pu  SaturateOnIntegerOverflow=on  OutDataTypeStr=Inherit: Same as input  ParamDataTypeStr=Inherit: Same as input
  Rtot_pu5 : Gain  Gain=Rtot_pu  SaturateOnIntegerOverflow=on  OutDataTypeStr=Inherit: Same as input  ParamDataTypeStr=Inherit: Same as input
  Saturation : Saturate  UpperLimit=2  LowerLimit=-2
  Sum : Sum  Inputs=|-+
  VdVq_conv : Outport
  wires:
  Mux/1 -> PI_Ireg1/1, Add2/2
  PI/1 -> Add2/1  "PI"
  Sum/1 -> PI/1
  IdIq_ref/1 -> Sum/2, Demux1/1
  IdIq_mes/1 -> Sum/1
  Add2/1 -> Saturation/1
  Saturation/1 -> VdVq_conv/1
  VdVq_mes/1 -> Demux/1
  Demux/1 -> Add1/1
  Rtot_pu1/1 -> Add1/2
  Demux1/1 -> Rtot_pu1/1, Ltot_pu2/1
  Ltot_pu1/1 -> Add1/3
  Demux1/2 -> Ltot_pu1/1, Rtot_pu5/1
  Rtot_pu5/1 -> Add3/2
  Ltot_pu2/1 -> Add3/3
  Add1/1 -> Mux/1  "Feedforward"
  Demux/2 -> Add3/1
  Add3/1 -> Mux/2

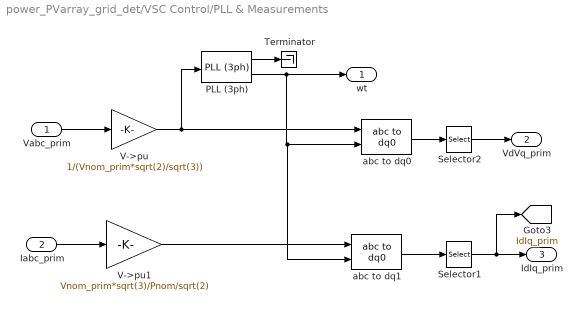
== system power_PVarray_grid_det/VSC Control/PLL & Measurements ==
  Vabc_prim : Inport
  Iabc_prim : Inport  Port=2
  PLL (3ph) : powerlib_meascontrol/PLL/PLL (3ph)  Fmin=45  Par_Init="[-0.57  Fnom]"  ParK=[180, 3200, 1]  TcD=1e-4  MaxRateChangeFreq=12  FilterCutOffFreq=25  Ts=Ts  AGC=on
  Selector1 : Selector  InputPortWidth=3  IndexOptions=Index vector (dialog)  Indices=[1 2]  OutputSizes=1
  Selector2 : Selector  InputPortWidth=3  IndexOptions=Index vector (dialog)  Indices=[1 2]  OutputSizes=1
  Terminator : Terminator
  V->pu : Gain  Gain=1/(Vnom_prim*sqrt(2)/sqrt(3))  SaturateOnIntegerOverflow=on  OutDataTypeStr=Inherit: Same as input  ParamDataTypeStr=Inherit: Same as input
  V->pu1 : Gain  Gain=Vnom_prim*sqrt(3)/Pnom/sqrt(2)  SaturateOnIntegerOverflow=on  OutDataTypeStr=Inherit: Same as input  ParamDataTypeStr=Inherit: Same as input
  abc to dq0 : powerlib_meascontrol/Transformations/abc to dq0  Alignment=90 degrees behind phase A axis
  abc to dq1 : powerlib_meascontrol/Transformations/abc to dq0  Alignment=90 degrees behind phase A axis
  wt : Outport
  VdVq_prim : Outport  Port=2
  IdIq_prim : Outport  Port=3
  tag scope: IdIq_prim=global
  wires:
  V->pu1/1 -> abc to dq1/1
  V->pu/1 -> PLL (3ph)/1, abc to dq0/1
  abc to dq1/1 -> Selector1/1
  Vabc_prim/1 -> V->pu/1
  Iabc_prim/1 -> V->pu1/1
  abc to dq0/1 -> Selector2/1
  Selector2/1 -> VdVq_prim/1
  Selector1/1 -> [IdIq_prim], IdIq_prim/1
  PLL (3ph)/2 -> wt/1, abc to dq1/2, abc to dq0/2
  PLL (3ph)/1 -> Terminator/1

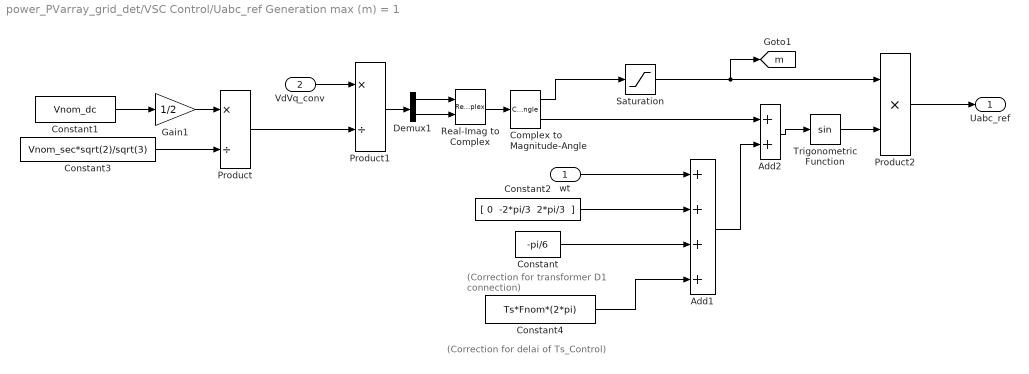
== system power_PVarray_grid_det/VSC Control/Uabc_ref Generation max (m) = 1 ==
  note: (Correction for transformer
      |  D1 connection)
  note: (Correction for delai of Ts_Control)
  wt : Inport
  VdVq_conv : Inport  Port=2
  Add1 : Sum  Inputs=++++
  Add2 : Sum
  Complex to Magnitude-Angle : ComplexToMagnitudeAngle
  Constant : Constant  Value=-pi/6
  Constant1 : Constant  Value=Vnom_dc
  Constant2 : Constant  Value="[ 0  -2*pi/3  2*pi/3  ]"
  Constant3 : Constant  Value=Vnom_sec*sqrt(2)/sqrt(3)
  Constant4 : Constant  Value=Ts*Fnom*(2*pi)
  Demux1 : Demux  Outputs=2
  Gain1 : Gain  Gain=1/2
  Product : Product  Inputs=*/  RndMeth=Zero
  Product1 : Product  Inputs=*/  RndMeth=Zero
  Product2 : Product  Inputs=**  RndMeth=Zero
  Real-Imag to Complex : RealImagToComplex
  Saturation : Saturate  UpperLimit=1  LowerLimit=0
  Trigonometric Function : Trigonometry
  Uabc_ref : Outport
  tag scope: m=global
  wires:
  Complex to Magnitude-Angle/1 -> Saturation/1
  Constant1/1 -> Gain1/1
  VdVq_conv/1 -> Product1/1
  Product1/1 -> Demux1/1
  Gain1/1 -> Product/1
  Real-Imag to Complex/1 -> Complex to Magnitude-Angle/1
  Demux1/1 -> Real-Imag to Complex/1
  Demux1/2 -> Real-Imag to Complex/2
  Constant2/1 -> Add1/2
  Constant/1 -> Add1/3
  Constant3/1 -> Product/2
  Product/1 -> Product1/2
  Complex to Magnitude-Angle/2 -> Add2/1
  Add1/1 -> Add2/2
  Add2/1 -> Trigonometric Function/1
  Saturation/1 -> [m], Product2/1
  Trigonometric Function/1 -> Product2/2
  Product2/1 -> Uabc_ref/1
  wt/1 -> Add1/1
  Constant4/1 -> Add1/4
